simulink model "THEOV_HW"  (R2018b)
settings: Solver=ode45  StartTime=0.0  StopTime=5  RelTol=1e-3  AbsTol=1e-6
PreLoadFcn:
  | % aeroblk_init_HL20
  | aero_guid_dat
StopFcn:
  | aero_guid_plot
undefined symbols (not defined in the file): alpha_ini, alpha_vec_Cn0, b_ref, Beamwidth, beta_vec_Cn0, Clbeta, Clda, Clddf, Cldr, Clp, Clr, Cm0, Cm_el, Cm_q, Cmda, Cmde, Cmdfn, Cmdfp, Cmdr, Cmq, Cn0, Cnda, Cnddf, Cndr, Cnp, Cnr, CX0, CXda, CXddf, CXde, CXdfn, CXdfp, CXdr, CYbeta, CYda, CYddf, CYdr, CZ0, Cz_el, CZda, CZde, CZdfn, CZdfp, CZdr, d2r, d_ref, g, h_ini, Iyy, K_r, Ks, l_acc, m2ft, mass, max_acc, max_gimbal, min_gimbal, pos_tgt, q_ini, S_ref ... (+8)
libraries: simulink_need_slupdate x10, aerospace x6, aeroblk_lib_HL20 x3, aerolibconvert2 x1, shared6dof x1, aerolibactuator x1, simulink x1
(part 2 of 2)

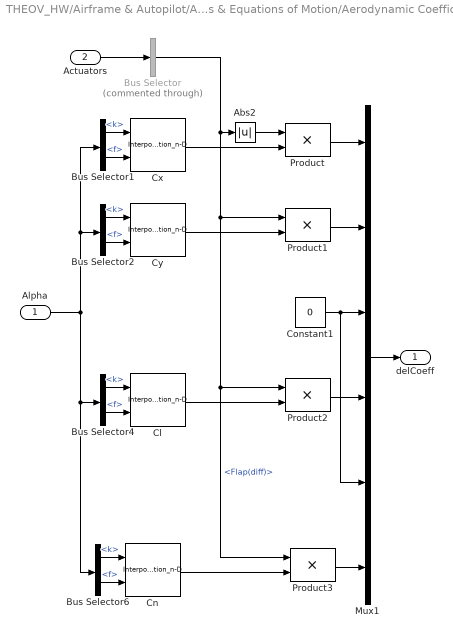
== system THEOV_HW/Airframe & Autopilot/Aerodynamics & Equations of Motion/Aerodynamic Coefficients/Actuator Increments/Flap(diff) ==
  Alpha : Inport
  Actuators : Inport  Port=2
  Abs2 : Abs  SaturateOnIntegerOverflow=on
  Bus Selector : BusSelector  Commented=through  OutputSignals=Flap(diff)
  Bus Selector{1..2,4,6} (4 alike) : BusSelector  OutputSignals=k,f
  Cl : Interpolation_n-D  NumberOfTableDimensions=1  Table=Clddf  RemoveProtectionIndex=on
      settings: InputPortMap=u0,u1
  Cn : Interpolation_n-D  NumberOfTableDimensions=1  Table=Cnddf  RemoveProtectionIndex=on
      settings: InputPortMap=u0,u1
  Constant1 : Constant  Value=0
  Cx : Interpolation_n-D  NumberOfTableDimensions=1  Table=CXddf  RemoveProtectionIndex=on
      settings: InputPortMap=u0,u1
  Cy : Interpolation_n-D  NumberOfTableDimensions=1  Table=CYddf  RemoveProtectionIndex=on
      settings: InputPortMap=u0,u1
  Mux1 : Mux  Inputs=6
  Product{,1..3} (4 alike) : Product  SaturateOnIntegerOverflow=on  InputSameDT=on  OutDataTypeStr=Inherit: Same as first input
  delCoeff : Outport
  wires:
  Bus Selector6/2 -> Cn/2  "<f>"
  Bus Selector6/1 -> Cn/1  "<k>"
  Bus Selector4/2 -> Cl/2  "<f>"
  Bus Selector4/1 -> Cl/1  "<k>"
  Bus Selector2/2 -> Cy/2  "<f>"
  Bus Selector2/1 -> Cy/1  "<k>"
  Bus Selector1/2 -> Cx/2  "<f>"
  Bus Selector1/1 -> Cx/1  "<k>"
  Constant1/1 -> Mux1/5, Mux1/3
  Abs2/1 -> Product/1
  Cn/1 -> Product3/2
  Product3/1 -> Mux1/6
  Cy/1 -> Product1/2
  Cl/1 -> Product2/2
  Product2/1 -> Mux1/4
  Product1/1 -> Mux1/2
  Bus Selector/1 -> Abs2/1, Product3/1, Product2/1, Product1/1  "<Flap(diff)>"
  Cx/1 -> Product/2
  Product/1 -> Mux1/1
  Actuators/1 -> Bus Selector/1
  Alpha/1 -> Bus Selector2/1, Bus Selector1/1, Bus Selector6/1, Bus Selector4/1
  Mux1/1 -> delCoeff/1

== system THEOV_HW/Airframe & Autopilot/Aerodynamics & Equations of Motion/Aerodynamic Coefficients/Actuator Increments/Flap(neg) ==
  Alpha : Inport
  Actuators : Inport  Port=2
  Bus Selector : BusSelector  Commented=through  OutputSignals=Flap(neg)
  Bus Selector1 : BusSelector  OutputSignals=k,f
  Bus Selector3 : BusSelector  OutputSignals=k,f
  Bus Selector5 : BusSelector  OutputSignals=k,f
  Cm : Interpolation_n-D  NumberOfTableDimensions=1  Table=Cmdfn  RemoveProtectionIndex=on
      settings: InputPortMap=u0,u1
  Constant1 : Constant  Value=0
  Constant2 : Constant  Value=0
  Constant3 : Constant  Value=0
  Cx : Interpolation_n-D  NumberOfTableDimensions=1  Table=CXdfn  RemoveProtectionIndex=on
      settings: InputPortMap=u0,u1
  Cz : Interpolation_n-D  NumberOfTableDimensions=1  Table=CZdfn  RemoveProtectionIndex=on
      settings: InputPortMap=u0,u1
  Mux1 : Mux  Inputs=6
  Product : Product  SaturateOnIntegerOverflow=on  InputSameDT=on  OutDataTypeStr=Inherit: Same as first input
  delCoeff : Outport
  wires:
  Bus Selector1/2 -> Cx/2  "<f>"
  Bus Selector1/1 -> Cx/1  "<k>"
  Bus Selector3/2 -> Cz/2  "<f>"
  Bus Selector3/1 -> Cz/1  "<k>"
  Bus Selector5/2 -> Cm/2  "<f>"
  Bus Selector5/1 -> Cm/1  "<k>"
  Bus Selector/1 -> Product/2  "<Flap(neg)>"
  Constant3/1 -> Mux1/6
  Constant2/1 -> Mux1/4
  Constant1/1 -> Mux1/2
  Actuators/1 -> Bus Selector/1
  Product/1 -> delCoeff/1
  Mux1/1 -> Product/1
  Alpha/1 -> Bus Selector1/1, Bus Selector3/1, Bus Selector5/1
  Cx/1 -> Mux1/1
  Cz/1 -> Mux1/3
  Cm/1 -> Mux1/5

== system THEOV_HW/Airframe & Autopilot/Aerodynamics & Equations of Motion/Aerodynamic Coefficients/Actuator Increments/Flap(pos) ==
  Alpha : Inport
  Actuators : Inport  Port=2
  Bus Selector : BusSelector  Commented=through  OutputSignals=Flap(pos)
  Bus Selector1 : BusSelector  OutputSignals=k,f
  Bus Selector3 : BusSelector  OutputSignals=k,f
  Bus Selector5 : BusSelector  OutputSignals=k,f
  Cm : Interpolation_n-D  NumberOfTableDimensions=1  Table=Cmdfp  RemoveProtectionIndex=on
      settings: InputPortMap=u0,u1
  Constant1 : Constant  Value=0
  Constant2 : Constant  Value=0
  Constant3 : Constant  Value=0
  Cx : Interpolation_n-D  NumberOfTableDimensions=1  Table=CXdfp  RemoveProtectionIndex=on
      settings: InputPortMap=u0,u1
  Cz : Interpolation_n-D  NumberOfTableDimensions=1  Table=CZdfp  RemoveProtectionIndex=on
      settings: InputPortMap=u0,u1
  Mux1 : Mux  Inputs=6
  Product : Product  SaturateOnIntegerOverflow=on  InputSameDT=on  OutDataTypeStr=Inherit: Same as first input
  delCoeff : Outport
  wires:
  Bus Selector1/2 -> Cx/2  "<f>"
  Bus Selector1/1 -> Cx/1  "<k>"
  Bus Selector3/2 -> Cz/2  "<f>"
  Bus Selector3/1 -> Cz/1  "<k>"
  Bus Selector5/2 -> Cm/2  "<f>"
  Bus Selector5/1 -> Cm/1  "<k>"
  Bus Selector/1 -> Product/2  "<Flap(pos)>"
  Actuators/1 -> Bus Selector/1
  Constant3/1 -> Mux1/6
  Constant2/1 -> Mux1/4
  Constant1/1 -> Mux1/2
  Cm/1 -> Mux1/5
  Cz/1 -> Mux1/3
  Cx/1 -> Mux1/1
  Alpha/1 -> Bus Selector1/1, Bus Selector3/1, Bus Selector5/1
  Mux1/1 -> Product/1
  Product/1 -> delCoeff/1

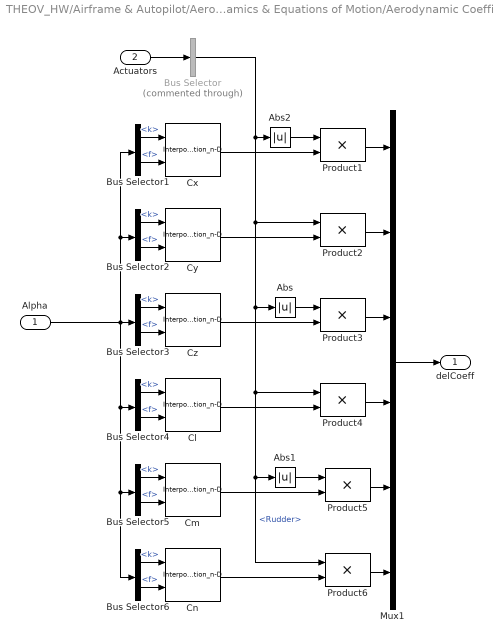
== system THEOV_HW/Airframe & Autopilot/Aerodynamics & Equations of Motion/Aerodynamic Coefficients/Actuator Increments/Rudder ==
  Alpha : Inport
  Actuators : Inport  Port=2
  Abs : Abs  SaturateOnIntegerOverflow=on
  Abs1 : Abs  SaturateOnIntegerOverflow=on
  Abs2 : Abs  SaturateOnIntegerOverflow=on
  Bus Selector : BusSelector  Commented=through  OutputSignals=Rudder
  Bus Selector{1..6} (6 alike) : BusSelector  OutputSignals=k,f
  Cl : Interpolation_n-D  NumberOfTableDimensions=1  Table=Cldr  RemoveProtectionIndex=on
      settings: InputPortMap=u0,u1
  Cm : Interpolation_n-D  NumberOfTableDimensions=1  Table=Cmdr  RemoveProtectionIndex=on
      settings: InputPortMap=u0,u1
  Cn : Interpolation_n-D  NumberOfTableDimensions=1  Table=Cndr  RemoveProtectionIndex=on
      settings: InputPortMap=u0,u1
  Cx : Interpolation_n-D  NumberOfTableDimensions=1  Table=CXdr  RemoveProtectionIndex=on
      settings: InputPortMap=u0,u1
  Cy : Interpolation_n-D  NumberOfTableDimensions=1  Table=CYdr  RemoveProtectionIndex=on
      settings: InputPortMap=u0,u1
  Cz : Interpolation_n-D  NumberOfTableDimensions=1  Table=CZdr  RemoveProtectionIndex=on
      settings: InputPortMap=u0,u1
  Mux1 : Mux  Inputs=6
  Product{1..6} (6 alike) : Product  SaturateOnIntegerOverflow=on  InputSameDT=on  OutDataTypeStr=Inherit: Same as first input
  delCoeff : Outport
  wires:
  Bus Selector6/2 -> Cn/2  "<f>"
  Bus Selector6/1 -> Cn/1  "<k>"
  Bus Selector5/2 -> Cm/2  "<f>"
  Bus Selector5/1 -> Cm/1  "<k>"
  Bus Selector4/2 -> Cl/2  "<f>"
  Bus Selector4/1 -> Cl/1  "<k>"
  Bus Selector3/2 -> Cz/2  "<f>"
  Bus Selector3/1 -> Cz/1  "<k>"
  Bus Selector2/2 -> Cy/2  "<f>"
  Bus Selector2/1 -> Cy/1  "<k>"
  Bus Selector1/2 -> Cx/2  "<f>"
  Bus Selector1/1 -> Cx/1  "<k>"
  Alpha/1 -> Bus Selector1/1, Bus Selector2/1, Bus Selector5/1, Bus Selector6/1, Bus Selector4/1, Bus Selector3/1
  Abs2/1 -> Product1/1
  Abs1/1 -> Product5/1
  Abs/1 -> Product3/1
  Bus Selector/1 -> Product6/1, Abs1/1, Product4/1, Abs/1, Product2/1, Abs2/1  "<Rudder>"
  Product6/1 -> Mux1/6
  Cn/1 -> Product6/2
  Product5/1 -> Mux1/5
  Cm/1 -> Product5/2
  Product4/1 -> Mux1/4
  Cl/1 -> Product4/2
  Cz/1 -> Product3/2
  Product3/1 -> Mux1/3
  Cy/1 -> Product2/2
  Product2/1 -> Mux1/2
  Cx/1 -> Product1/2
  Product1/1 -> Mux1/1
  Mux1/1 -> delCoeff/1
  Actuators/1 -> Bus Selector/1

== system THEOV_HW/Airframe & Autopilot/Aerodynamics & Equations of Motion/Aerodynamic Coefficients/Body Rate Damping/p ==
  Alpha : Inport
  Bus Selector : BusSelector  OutputSignals=k,f
  Bus Selector1 : BusSelector  OutputSignals=k,f
  Cl : Interpolation_n-D  NumberOfTableDimensions=1  Table=Clp  RemoveProtectionIndex=on
      settings: InputPortMap=u0,u1
  Cn : Interpolation_n-D  NumberOfTableDimensions=1  Table=Cnp  RemoveProtectionIndex=on
      settings: InputPortMap=u0,u1
  Constant1 : Constant  Value=0
  Mux1 : Mux  Inputs=6
  delCoeff : Outport
  wires:
  Bus Selector1/2 -> Cn/2  "<f>"
  Bus Selector1/1 -> Cn/1  "<k>"
  Bus Selector/2 -> Cl/2  "<f>"
  Bus Selector/1 -> Cl/1  "<k>"
  Alpha/1 -> Bus Selector1/1, Bus Selector/1
  Cl/1 -> Mux1/4  "Cl"
  Cn/1 -> Mux1/6
  Constant1/1 -> Mux1/2, Mux1/3, Mux1/5, Mux1/1  "Cxp"
  Mux1/1 -> delCoeff/1

== system THEOV_HW/Airframe & Autopilot/Aerodynamics & Equations of Motion/Aerodynamic Coefficients/Body Rate Damping/q ==
  Alpha : Inport
  Bus Selector1 : BusSelector  OutputSignals=k,f
  Cmq : Interpolation_n-D  NumberOfTableDimensions=1  Table=Cmq  RemoveProtectionIndex=on
      settings: InputPortMap=u0,u1
  Constant3 : Constant  Value=0
  Mux1 : Mux  Inputs=6
  delCoeff : Outport
  wires:
  Bus Selector1/2 -> Cmq/2  "<f>"
  Bus Selector1/1 -> Cmq/1  "<k>"
  Alpha/1 -> Bus Selector1/1
  Mux1/1 -> delCoeff/1
  Constant3/1 -> Mux1/4, Mux1/6, Mux1/3, Mux1/2, Mux1/1
  Cmq/1 -> Mux1/5

== system THEOV_HW/Airframe & Autopilot/Aerodynamics & Equations of Motion/Aerodynamic Coefficients/Body Rate Damping/r ==
  Alpha : Inport
  Bus Selector : BusSelector  OutputSignals=k,f
  Bus Selector1 : BusSelector  OutputSignals=k,f
  Cl : Interpolation_n-D  NumberOfTableDimensions=1  Table=Clr  RemoveProtectionIndex=on
      settings: InputPortMap=u0,u1
  Cn : Interpolation_n-D  NumberOfTableDimensions=1  Table=Cnr  RemoveProtectionIndex=on
      settings: InputPortMap=u0,u1
  Constant : Constant  Value=0
  Mux1 : Mux  Inputs=6
  delCoeff : Outport
  wires:
  Bus Selector1/2 -> Cn/2  "<f>"
  Bus Selector1/1 -> Cn/1  "<k>"
  Bus Selector/2 -> Cl/2  "<f>"
  Bus Selector/1 -> Cl/1  "<k>"
  Alpha/1 -> Bus Selector/1, Bus Selector1/1
  Mux1/1 -> delCoeff/1
  Constant/1 -> Mux1/3, Mux1/5, Mux1/2, Mux1/1  "Cxr"
  Cl/1 -> Mux1/4  "Cl"
  Cn/1 -> Mux1/6

== system THEOV_HW/Airframe & Autopilot/Aerodynamics & Equations of Motion/Aerodynamic Coefficients/missile_coeff/Fins ==
  Fin : Inport
  Cm : Gain  Gain=Cm_el  SaturateOnIntegerOverflow=on  OutDataTypeStr=Inherit: Same as input  ParamDataTypeStr=Inherit: Same as input
  Cx : Gain  Gain=0  SaturateOnIntegerOverflow=on  OutDataTypeStr=Inherit: Same as input  ParamDataTypeStr=Inherit: Same as input
  Cz : Gain  Gain=Cz_el  SaturateOnIntegerOverflow=on  OutDataTypeStr=Inherit: Same as input  ParamDataTypeStr=Inherit: Same as input
  Cx_el : Outport  InitialOutput=0
  Cz_el : Outport  Port=2  InitialOutput=0
  Cm_el : Outport  Port=3  InitialOutput=0
  wires:
  Fin/1 -> Cx/1, Cm/1, Cz/1
  Cx/1 -> Cx_el/1
  Cm/1 -> Cm_el/1
  Cz/1 -> Cz_el/1

== system THEOV_HW/Airframe & Autopilot/Aerodynamics & Equations of Motion/Aerodynamic Coefficients/missile_coeff/Incidence ==
  Mach : Inport
  Alpha : Inport  Port=2
  Alpha Index : simulink_need_slupdate/PreLookup Index Search  bpData=alpha_vec  searchMode=Binary Search  cacheBpFlag=on  outputFlag=off  IndexDataType=uint32  extrapMode=Linear Extrapolation  rangeErrorMode=None
      settings: SourceProductName=Simulink  SourceProductBaseCode=SL
  Cm : simulink_need_slupdate/Interpolation (n-D) using PreLookup  numDimsPopupSelect=2  explicitNumDims=2  table=Cm_alpha  interpMethod=Linear  extrapMethod=Linear  rangeErrorMode=None  NumSelectionDims=0
      settings: SourceProductName=Simulink  SourceProductBaseCode=SL
  Cx : simulink_need_slupdate/Interpolation (n-D) using PreLookup  numDimsPopupSelect=2  explicitNumDims=2  table=Cx_alpha  interpMethod=Linear  extrapMethod=Linear  rangeErrorMode=None  NumSelectionDims=0
      settings: SourceProductName=Simulink  SourceProductBaseCode=SL
  Cz : simulink_need_slupdate/Interpolation (n-D) using PreLookup  numDimsPopupSelect=2  explicitNumDims=2  table=Cz_alpha  interpMethod=Linear  extrapMethod=Linear  rangeErrorMode=None  NumSelectionDims=0
      settings: SourceProductName=Simulink  SourceProductBaseCode=SL
  Mach Index : simulink_need_slupdate/PreLookup Index Search  bpData=Mach_vec  searchMode=Binary Search  cacheBpFlag=on  outputFlag=off  IndexDataType=uint32  extrapMode=Linear Extrapolation  rangeErrorMode=None
      settings: SourceProductName=Simulink  SourceProductBaseCode=SL
  Cx_alpha : Outport  InitialOutput=0
  Cz_alpha : Outport  Port=2  InitialOutput=0
  Cm_alpha : Outport  Port=3  InitialOutput=0
  wires:
  Alpha Index/1 -> Cx/1, Cz/1, Cm/1
  Mach Index/1 -> Cz/2, Cm/2, Cx/2
  Cx/1 -> Cx_alpha/1
  Cz/1 -> Cz_alpha/1
  Cm/1 -> Cm_alpha/1
  Alpha/1 -> Alpha Index/1
  Mach/1 -> Mach Index/1

== stateflow chart THEOV_HW/Guidance/Guidance Processor (Updated @100Hz) ==
  settings: updateMethod=DISCRETE  sampleTime=0.01
  state Guidance [parallel]
    settings: executionOrder=1
    state Target_Search
      en: Mode=1;Sigma_d=0;incr=-100;Acquire_time=t;
      du: Sigma_d=Sigma_d+0.01*incr;
      Target_Search -> Target_Search [order 1] : [Sigma_d>30||Sigma_d<-30]  / incr=-incr;
    state Target_Lock
      en:Mode=2;Acquire_time=t;
    state Abort
      en:Detonate=1;
    state Radar_Guided
      en:Mode=3;
      ex:az_fix=az_dem;
    state Blind_Range
      en:Mode=4;
    (default) -> Target_Search : {az_fix=-9.81;}
    Radar_Guided -> Target_Search [order 1] : [Acquire==0]
    Target_Search -> Abort [order 2] : [t-Acquire_time>7]
        | / send(Timeout, Fuze);
    Target_Search -> Target_Lock [order 1] : [Acquire==1]
    Target_Lock -> Radar_Guided : [t-Acquire_time>0.2]
    Radar_Guided -> Blind_Range [order 2] : [Range<200]
  state Fuze [parallel]
    settings: executionOrder=2
    state Armed
      en:Fuze=1;
    state Inert
      en:Fuze = 0;
    Inert -> Armed [order 2] : [in(Guidance.Radar_Guided)&&Range<1000]
    (default) -> Inert
    Inert -> Armed [order 1] : Timeout
    Armed -> Inert : enter(Guidance.Target_Search)
  data: Range input double; Detonate output boolean; Fuze output boolean; Sigma_d output double; Mode output uint8; Acquire input boolean; Acquire_time local double; incr local double; az_dem input double; az_fix output double =-9.81
  data Sigma_d settings: description=Demanded Seeker Look Angle
  data Acquire settings: description=Seeker Acquisition Flag
  data incr settings: description=Seeker Search Rate
  events: Timeout local EITHER_EDGE_EVENT

== matlab function THEOV_HW/Airframe & Autopilot/Aerodynamics & Equations of Motion/MATLAB Function ==
  data: DCMeb input; angular_rates_earth output; angular_rates_body input
function angular_rates_earth  = fcn(DCMeb, angular_rates_body)

angular_rates_earth = DCMeb.' * angular_rates_body;
